simulink model "polokwaneSIL"  (R2024a)
settings: Solver=FixedStepAuto  StartTime=0.0  StopTime=43200  FixedStep=60  MaxStep=60  RelTol=1e-3
InitFcn:
  | load("inputBusObj.mat");
settings Model: Creator=eunice.duplessis  LastModifiedBy=jason.miskin
settings DataIOCC: ExternalInput=slInputs  LoadExternalInput=on
settings DebuggingCC: AllowedUnitSystems=SI,SI (extended)

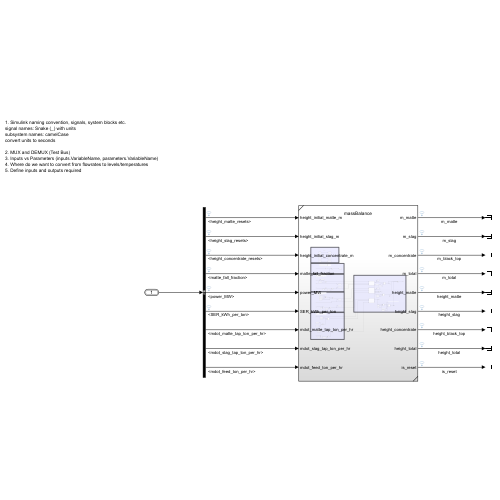
[thumbnail: Simulink's stored preview of the top-level diagram]
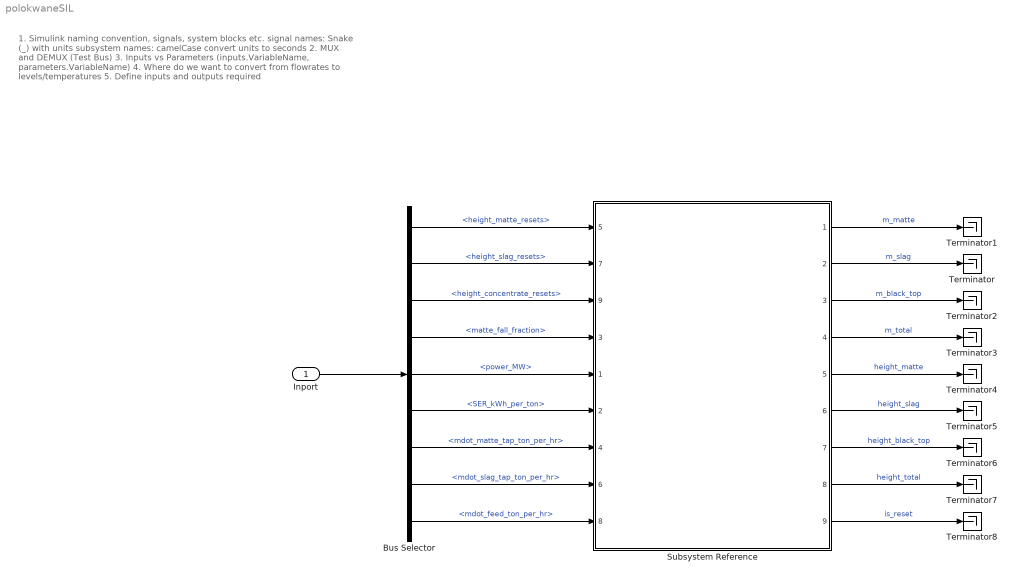
== system polokwaneSIL ==
  note: 1. Simulink naming convention, signals, system blocks etc.
      | signal names: Snake (_) with units
      | subsystem names: camelCase
      | convert units to seconds
      |
      | 2. MUX and DEMUX (Test Bus)
      | 3. Inputs vs Parameters (inputs.VariableName, parameters.VariableName)
      | 4. Where do we want to convert from flowrates to levels/temperatures
      | 5. Define inputs and outputs required
  Inport : Inport  OutDataTypeStr=Bus: inputs_busObj
  Bus Selector : BusSelector  OutputSignals=height_matte_resets,height_slag_resets,height_concentrate_resets,matte_fall_fraction,power_MW,SER_kWh_per_ton,mdot_matte_tap_ton_per_hr,mdot_slag_tap_ton_per_hr,mdot_feed_ton_per_hr
  Subsystem Reference : Subsystem  ReferencedSubsystem=massBalance
      settings: PermitHierarchicalResolution=None  PortSchema="{\"entries\":[{\"content\":{\"sides\":[{\"content\":{\"connectorIds\":[\"In5\",\"In7\",\"In9\",\"In3\",\"In1\",\"In2\",\"In4\",\"In6\",\"In8\"]},\"type\":\"ConnectorPlacement.EquallySpacedRectSide\",\"uuid\":\"2a3e936f-bd4d-49f5-bd7a-b038e806c339\"},{\"content\":{\"connectorIds\":[\"Out1\",\"Out2\",\"Out3\",\"Out4\",\"Out5\",\"Out6\",\"Out7\",\"Out8\",\"Out9\"],\"side\":\"RIGHT\"},\"type\":\"ConnectorPlacement.EquallySpacedRectSide\",\"uuid\":\"eb8ae07c-65a6-425b-bf63-6660ad54bf25\"},{\"content\":{\"side\":\"TOP\"},\"type\":\"ConnectorPlacement.EquallySpacedRectSide\",\"uuid\":\"98cc8c0b-63a0-45ed-8085-e14bfed4c114\"}]},\"type\":\"ConnectorPlacement.EquallySpacedConnector\",\"uuid\":\"84fa6f9e-9fac-4494-bdca-170a2db95ef2\"}],\"packageUris\":[\"http://schema.mathworks.com/mf0/Connector/R2020b\"],\"version\":\"1.0\"}"
  Terminator{,1..8} (9 alike) : Terminator
  wires:
  Inport/1 -> Bus Selector/1
  Bus Selector/9 -> Subsystem Reference/8  "<mdot_feed_ton_per_hr>"
  Bus Selector/8 -> Subsystem Reference/6  "<mdot_slag_tap_ton_per_hr>"
  Bus Selector/7 -> Subsystem Reference/4  "<mdot_matte_tap_ton_per_hr>"
  Bus Selector/4 -> Subsystem Reference/3  "<matte_fall_fraction>"
  Bus Selector/6 -> Subsystem Reference/2  "<SER_kWh_per_ton>"
  Bus Selector/5 -> Subsystem Reference/1  "<power_MW>"
  Subsystem Reference/1 -> Terminator1/1  "m_matte"
  Subsystem Reference/3 -> Terminator2/1  "m_black_top"
  Subsystem Reference/4 -> Terminator3/1  "m_total"
  Subsystem Reference/5 -> Terminator4/1  "height_matte"
  Subsystem Reference/6 -> Terminator5/1  "height_slag"
  Subsystem Reference/7 -> Terminator6/1  "height_black_top"
  Subsystem Reference/8 -> Terminator7/1  "height_total"
  Subsystem Reference/2 -> Terminator/1  "m_slag"
  Bus Selector/1 -> Subsystem Reference/5  "<height_matte_resets>"
  Bus Selector/2 -> Subsystem Reference/7  "<height_slag_resets>"
  Bus Selector/3 -> Subsystem Reference/9  "<height_concentrate_resets>"
  Subsystem Reference/9 -> Terminator8/1  "is_reset"
